simulink model "Perreault2004"  (R2018a)
settings: Solver=VariableStepAuto  StartTime=0  StopTime=0.05  FixedStep=1e-6
undefined symbols (not defined in the file): alternator, electrical_load, rectifier, T_k, T_s
libraries: elec_lib x26, fl_lib x25, nesl_utility x24, SimscapeCustomBlocks_lib x2, simulink x2
(part 2 of 2)

== matlab function Perreault2004/Load Matching Switched-Mode Rectifier Controller/MATLAB Function ==
  data: n_r input; u_smr output; i_f input; p input; v_o input; u_lim_l input; u_lim_u input
function u_smr = load_matching_smr_controller(n_r, i_f, p, v_o, u_lim_l, u_lim_u)

epsilon = 1e-3;

if (i_f < epsilon)
    u_smr = 0;
else
    k_e = 0;
    
    omega_r = 2*pi*n_r/60;
    omega_e = p*omega_r;
    u_smr = 1 - ((sqrt(2)*pi*k_e)/(4*v_o))*omega_e*i_f;
%     u_smr = 1 - ((3*sqrt(3)/pi)*(k_e*omega_a*i_f)/v_o);
    
    if (u_smr > u_lim_u)
        u_smr = u_lim_u;
    elseif (u_smr < u_lim_l)
        u_smr = u_lim_l;
    end
end

end
